simulink model "PNG_guidanceloop"  (R2019b)
settings: Solver=VariableStepAuto  StartTime=0.0  StopTime=9.998  RelTol=1e-3
settings Model: Creator=win10  LastModifiedBy=win10

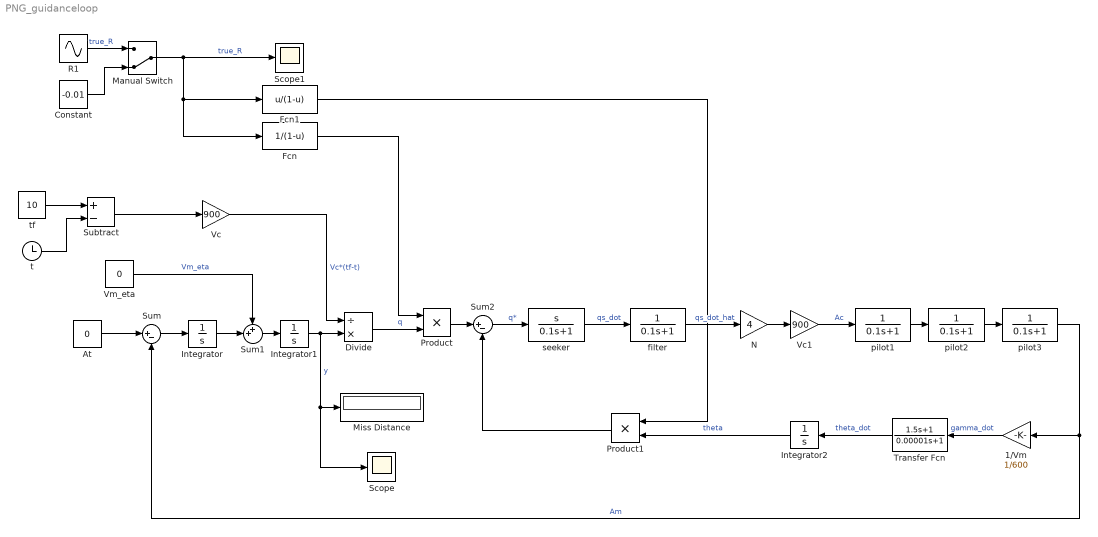
== system PNG_guidanceloop ==
  1/Vm : Gain  Gain=1/600
  At : Constant  Value=0
  Constant : Constant  Value=-0.01
  Divide : Product  Inputs=/*
  Fcn : Fcn  Expr=1/(1-u)
  Fcn1 : Fcn  Expr=u/(1-u)
  Integrator : Integrator  InitialCondition=900
  Integrator1 : Integrator  InitialCondition=20
  Integrator2 : Integrator
  Manual Switch : ManualSwitch  CurrentSetting=0
  Miss Distance : Display
  N : Gain  Gain=4
  Product : Product
  Product1 : Product
  R1 : Sin  Amplitude=0.06  Frequency=pi/2  SampleTime=0
  Scope : Scope
  Scope1 : Scope
  Subtract : Sum  Inputs=+-
  Sum : Sum  Inputs=|+-
  Sum1 : Sum  Inputs=++|
  Sum2 : Sum  Inputs=|+-
  Transfer Fcn : TransferFcn  Numerator=[1.5 1]  Denominator=[0.00001 1]
  Vc : Gain  Gain=900
  Vc1 : Gain  Gain=900
  Vm_eta : Constant  Value=0
  filter : TransferFcn  Denominator=[0.1 1]
  pilot1 : TransferFcn  Denominator=[0.1 1]
  pilot2 : TransferFcn  Denominator=[0.1 1]
  pilot3 : TransferFcn  Denominator=[0.1 1]
  seeker : TransferFcn  Numerator=[1 0]  Denominator=[0.1 1]
  t : Clock
  tf : Constant  Value=10
  wires:
  tf/1 -> Subtract/1
  At/1 -> Sum/1
  Integrator/1 -> Sum1/2
  Sum1/1 -> Integrator1/1
  t/1 -> Subtract/2
  Vm_eta/1 -> Sum1/1  "Vm_eta"
  Subtract/1 -> Vc/1
  Vc/1 -> Divide/1  "Vc*(tf-t)"
  Integrator1/1 -> Miss Distance/1, Scope/1, Divide/2  "y"
  Sum/1 -> Integrator/1
  pilot2/1 -> pilot3/1
  filter/1 -> N/1  "qs_dot_hat"
  Constant/1 -> Manual Switch/2
  Manual Switch/1 -> Scope1/1, Fcn1/1, Fcn/1  "true_R"
  Product/1 -> Sum2/1
  Transfer Fcn/1 -> Integrator2/1  "theta_dot"
  Integrator2/1 -> Product1/2  "theta"
  Product1/1 -> Sum2/2
  Sum2/1 -> seeker/1  "q*"
  Vc1/1 -> pilot1/1  "Ac"
  1/Vm/1 -> Transfer Fcn/1  "gamma_dot"
  N/1 -> Vc1/1
  R1/1 -> Manual Switch/1  "true_R"
  seeker/1 -> filter/1  "qs_dot"
  pilot1/1 -> pilot2/1
  pilot3/1 -> Sum/2, 1/Vm/1  "Am"
  Fcn1/1 -> Product1/1
  Fcn/1 -> Product/1
  Divide/1 -> Product/2  "q"
